simulink model "UDP_server"  (R2019b)
settings: Solver=VariableStepAuto  StartTime=0.0  StopTime=inf  RelTol=1e-3
libraries: dspnetwork x2
settings Model: Creator=maxime  LastModifiedBy=maxime

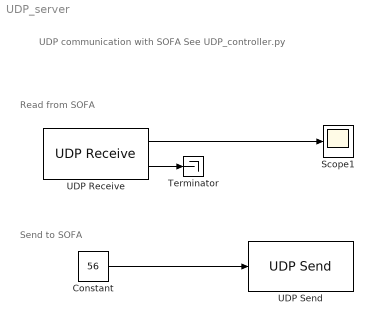
== system UDP_server ==
  note: Send to SOFA
  note: Read from SOFA
  note: UDP communication with SOFA
      | See UDP_controller.py
  Constant : Constant  Value=56
  Scope1 : Scope
  Terminator : Terminator
  UDP Receive : dspnetwork/UDP Receive  localURL='0.0.0.0'  localPort=5006  remoteURL='127.0.0.1'  remotePort=-1  recvBufferSize=1  dims=1  signalDatatype=double  isComplex=off  isVarSize=off  showBlockingTime=off  blockingTime=0  sampletime=1  blockPlatform=[]
      settings: SourceProductName=Simulink
  UDP Send : dspnetwork/UDP Send  remoteURL='127.0.0.1'  remotePort=5005  localURL='0.0.0.0'  localPortSource=Automatically determine  localPort=-1  sampletime=-1  blockPlatform=[]  separateLengthPort=0
      settings: SourceProductName=Simulink
  wires:
  UDP Receive/1 -> Scope1/1
  Constant/1 -> UDP Send/1
  UDP Receive/2 -> Terminator/1
